simulink library "myblocksets"  (Simulink 6.3)
settings Model: LastModifiedBy=sangwook

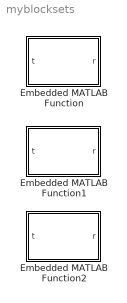
== system myblocksets ==
  Embedded MATLAB Function : Stateflow chart
  Embedded MATLAB Function1 : Stateflow chart
  Embedded MATLAB Function2 : Stateflow chart

== matlab function Embedded MATLAB Function1 ==
  data: t input inherited; r output inherited
%ROTY Rotation about Y axis
%
%	TR = ROTY(theta)
%
% Returns a homogeneous transformation representing a rotation of theta 
% about the Y axis.
%
% See also: ROTX, ROTZ, ROTVEC.

% $Log: roty.m,v $
% Revision 1.2  2002/04/01 11:47:16  pic
% General cleanup of code: help comments, see also, copyright, remnant dh/dyn
% references, clarification of functions.
%
% $Revision: 1.2 $
% Copyright (C) 1993-2002, by Peter I. Corke

function r = roty(t)
	ct = cos(t);
	st = sin(t);
	r =    [ct	0	st	0
		0	1	0	0
		-st	0	ct	0
		0	0	0	1];

== matlab function Embedded MATLAB Function ==
  data: t input inherited; r output inherited
%ROTX Rotation about X axis
%
%	TR = ROTX(theta)
%
% Returns a homogeneous transformation representing a rotation of theta 
% about the X axis.
%
% See also: ROTY, ROTZ, ROTVEC.

% $Log: rotx.m,v $
% Revision 1.2  2002/04/01 11:47:16  pic
% General cleanup of code: help comments, see also, copyright, remnant dh/dyn
% references, clarification of functions.
%
% $Revision: 1.2 $
% Copyright (C) 1993-2002, by Peter I. Corke

function r = rotx(t)
	ct = cos(t);
	st = sin(t);
	r =    [1	0	0	0
		0	ct	-st	0
		0	st	ct	0
		0	0	0	1];

== matlab function Embedded MATLAB Function2 ==
  data: t input inherited; r output inherited
%ROTZ Rotation about Z axis
%
%	TR = ROTZ(theta)
%
% Returns a homogeneous transformation representing a rotation of theta 
% about the Z axis.
%
% See also: ROTX, ROTY, ROTVEC.

% $Log: rotz.m,v $
% Revision 1.2  2002/04/01 11:47:16  pic
% General cleanup of code: help comments, see also, copyright, remnant dh/dyn
% references, clarification of functions.
%
% $Revision: 1.2 $
% Copyright (C) 1993-2002, by Peter I. Corke

function r = rotz(t)
	ct = cos(t);
	st = sin(t);
	r =    [ct	-st	0	0
		st	ct	0	0
		0	0	1	0
		0	0	0	1];
